simulink model "cdip_pdcont"  (R2013a)
settings: Solver=ode1  StartTime=0.0  StopTime=8  FixedStep=0.001  RelTol=1e-3
values from neighbouring files (symbols this model uses):
  dtheta_0 = 0    [cdip_lqr_servo_sim.m]    (also in cdip_lqr_sim.m; cdip_pdcont_sim.m)
  dz_0 = 0    [cdip_lqr_servo_sim.m]    (also in cdip_lqr_sim.m; cdip_pdcont_sim.m)
  kD = 0.75    [cdip_pdcont_sim.m]
  kP = 10    [cdip_pdcont_sim.m]
  theta_0 = 0    [cdip_lqr_servo_sim.m]    (also in cdip_lqr_sim.m = 0.261799387799; cdip_pdcont_sim.m = 3.14159265359)
  z_0 = 0    [cdip_lqr_servo_sim.m]    (also in cdip_lqr_sim.m; cdip_pdcont_sim.m)
undefined symbols (not defined in the file or in its folder): ac, bc, g, Jp, lp, mp, mup
settings Model: Creator=kawata  LastModifiedBy=kawata
settings DataIOCC: LimitDataPoints=off  SignalLoggingSaveFormat=ModelDataLogs
settings OptimizationCC: ExpressionDepthLimit=2147483647
settings DebuggingCC: FcnCallInpInsideContextMsg=UseLocalSettings
settings GRTTargetCC: CombineOutputUpdateFcns=off  GRTInterface=on

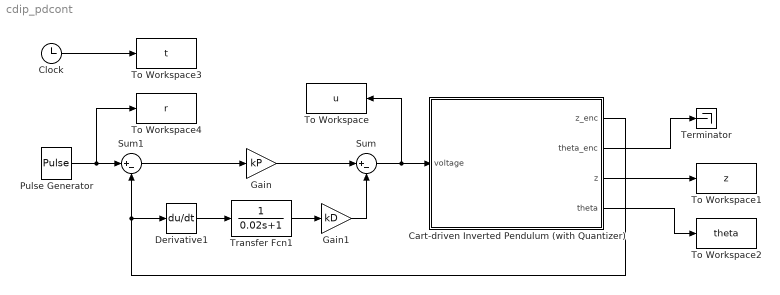
== system cdip_pdcont ==
  Cart-driven Inverted Pendulum (with Quantizer) : Subsystem
      mask Display: image(imread('cdip_photo.jpg'),'center')
  Clock : Clock
  Derivative1 : Derivative
  Gain : Gain  Gain=kP  SaturateOnIntegerOverflow=on  OutDataTypeStr=Inherit: Same as input  ParamDataTypeStr=Inherit: Same as input
  Gain1 : Gain  Gain=kD  SaturateOnIntegerOverflow=on  OutDataTypeStr=Inherit: Same as input  ParamDataTypeStr=Inherit: Same as input
  Pulse Generator : DiscretePulseGenerator  PulseType=Time based  Amplitude=0.4  Period=4  PulseWidth=50
  Sum : Sum  Inputs=|+-  SaturateOnIntegerOverflow=on  InputSameDT=on  OutDataTypeStr=Inherit: Same as first input
  Sum1 : Sum  Inputs=|+-  SaturateOnIntegerOverflow=on  InputSameDT=on  OutDataTypeStr=Inherit: Same as first input
  Terminator : Terminator
  To Workspace : ToWorkspace  VariableName=u  SampleTime=-1
  To Workspace1 : ToWorkspace  VariableName=z  SampleTime=-1
  To Workspace2 : ToWorkspace  VariableName=theta  SampleTime=-1
  To Workspace3 : ToWorkspace  VariableName=t  SampleTime=-1
  To Workspace4 : ToWorkspace  VariableName=r  SampleTime=-1
  Transfer Fcn1 : TransferFcn  Denominator=[0.02 1]
  wires:
  Pulse Generator/1 -> To Workspace4/1, Sum1/1
  Cart-driven Inverted Pendulum (with Quantizer)/4(theta) -> To Workspace2/1
  Clock/1 -> To Workspace3/1
  Gain/1 -> Sum/1
  Sum1/1 -> Gain/1
  Transfer Fcn1/1 -> Gain1/1
  Gain1/1 -> Sum/2
  Sum/1 -> Cart-driven Inverted Pendulum (with Quantizer)/1(voltage), To Workspace/1
  Derivative1/1 -> Transfer Fcn1/1
  Cart-driven Inverted Pendulum (with Quantizer)/1(z_enc) -> Derivative1/1, Sum1/2
  Cart-driven Inverted Pendulum (with Quantizer)/3(z) -> To Workspace1/1
  Cart-driven Inverted Pendulum (with Quantizer)/2(theta_enc) -> Terminator/1

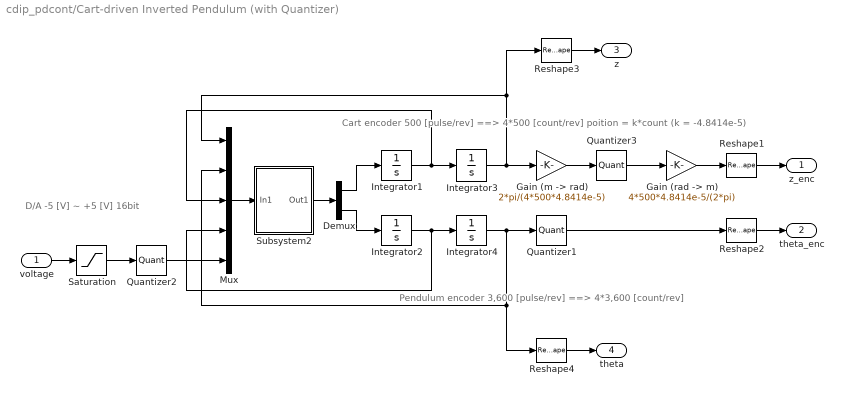
== system cdip_pdcont/Cart-driven Inverted Pendulum (with Quantizer) ==
  note: Cart encoder
      |   500 [pulse/rev]  ==> 4*500 [count/rev]
      |   poition = k*count  (k = -4.8414e-5)
  note: D/A
      |   -5 [V] ~ +5 [V]
      |  16bit
  note: Pendulum encoder
      |   3,600 [pulse/rev]  ==> 4*3,600 [count/rev]
  voltage : Inport
  Demux : Demux  Outputs=2
  "Gain (m -> rad)" : Gain  Gain=2*pi/(4*500*4.8414e-5)  SaturateOnIntegerOverflow=on  OutDataTypeStr=Inherit: Same as input  ParamDataTypeStr=Inherit: Same as input
  "Gain (rad -> m)" : Gain  Gain=4*500*4.8414e-5/(2*pi)  SaturateOnIntegerOverflow=on  OutDataTypeStr=Inherit: Same as input  ParamDataTypeStr=Inherit: Same as input
  Integrator1 : Integrator  InitialCondition=dz_0
  Integrator2 : Integrator  InitialCondition=dtheta_0
  Integrator3 : Integrator  InitialCondition=z_0
  Integrator4 : Integrator  InitialCondition=theta_0
  Mux : Mux  Inputs=5
  Quantizer1 : Quantizer  QuantizationInterval=2*pi/(4*3600)
  Quantizer2 : Quantizer  QuantizationInterval=10/2^(16)
  Quantizer3 : Quantizer  QuantizationInterval=2*pi/(4*500)
  Reshape{1..4} (4 alike) : Reshape
  Saturation : Saturate  UpperLimit=5  LowerLimit=-5
  Subsystem2 : Subsystem
  z_enc : Outport
  theta_enc : Outport  Port=2
  z : Outport  Port=3
  theta : Outport  Port=4
  wires:
  Reshape4/1 -> theta/1
  Reshape3/1 -> z/1
  Saturation/1 -> Quantizer2/1
  Quantizer2/1 -> Mux/5
  Quantizer1/1 -> Reshape2/1
  Subsystem2/1(Out1) -> Demux/1
  Mux/1 -> Subsystem2/1(In1)
  Demux/1 -> Integrator1/1
  Demux/2 -> Integrator2/1
  Integrator1/1 -> Mux/3, Integrator3/1
  Integrator2/1 -> Mux/4, Integrator4/1
  Integrator3/1 -> Reshape3/1, Mux/1, "Gain (m -> rad)"/1
  Integrator4/1 -> Reshape4/1, Mux/2, Quantizer1/1
  voltage/1 -> Saturation/1
  "Gain (m -> rad)"/1 -> Quantizer3/1
  Quantizer3/1 -> "Gain (rad -> m)"/1
  "Gain (rad -> m)"/1 -> Reshape1/1
  Reshape1/1 -> z_enc/1
  Reshape2/1 -> theta_enc/1

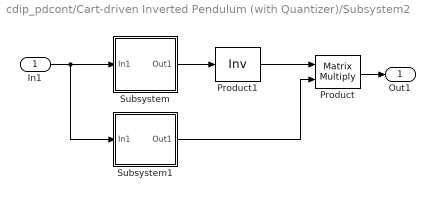
== system cdip_pdcont/Cart-driven Inverted Pendulum (with Quantizer)/Subsystem2 ==
  In1 : Inport
  Product : Product  Multiplication=Matrix(*)  SaturateOnIntegerOverflow=on  InputSameDT=on  OutDataTypeStr=Inherit: Same as first input
  Product1 : Product  Inputs=/  Multiplication=Matrix(*)  SaturateOnIntegerOverflow=on  InputSameDT=on  OutDataTypeStr=Inherit: Same as first input
  Subsystem : Subsystem
  Subsystem1 : Subsystem
  Out1 : Outport
  wires:
  Subsystem/1(Out1) -> Product1/1
  Product1/1 -> Product/1
  Subsystem1/1(Out1) -> Product/2
  In1/1 -> Subsystem/1(In1), Subsystem1/1(In1)
  Product/1 -> Out1/1

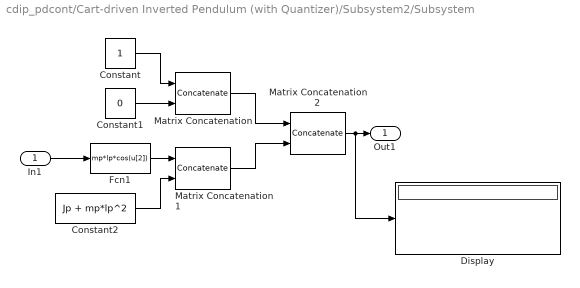
== system cdip_pdcont/Cart-driven Inverted Pendulum (with Quantizer)/Subsystem2/Subsystem ==
  In1 : Inport
  Constant : Constant
  Constant1 : Constant  Value=0
  Constant2 : Constant  Value=Jp + mp*lp^2
  Display : Display
  Fcn1 : Fcn  Expr=mp*lp*cos(u[2])
  Matrix Concatenation : Concatenate  Mode=Multidimensional array  ConcatenateDimension=2
  Matrix Concatenation1 : Concatenate  Mode=Multidimensional array  ConcatenateDimension=2
  Matrix Concatenation2 : Concatenate  Mode=Multidimensional array
  Out1 : Outport
  wires:
  Constant2/1 -> Matrix Concatenation1/2
  Fcn1/1 -> Matrix Concatenation1/1
  In1/1 -> Fcn1/1
  Matrix Concatenation/1 -> Matrix Concatenation2/1
  Matrix Concatenation1/1 -> Matrix Concatenation2/2
  Matrix Concatenation2/1 -> Display/1, Out1/1
  Constant/1 -> Matrix Concatenation/1
  Constant1/1 -> Matrix Concatenation/2

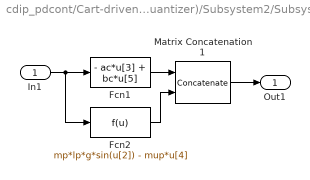
== system cdip_pdcont/Cart-driven Inverted Pendulum (with Quantizer)/Subsystem2/Subsystem1 ==
  In1 : Inport
  Fcn1 : Fcn  Expr=- ac*u[3] + bc*u[5]
  Fcn2 : Fcn  Expr=mp*lp*g*sin(u[2]) - mup*u[4]
  Matrix Concatenation1 : Concatenate  Mode=Multidimensional array
  Out1 : Outport
  wires:
  Fcn2/1 -> Matrix Concatenation1/2
  Fcn1/1 -> Matrix Concatenation1/1
  In1/1 -> Fcn2/1, Fcn1/1
  Matrix Concatenation1/1 -> Out1/1
